simulink model "STM32_IIR_test_script"  (R2018b)
settings: Solver=FixedStepAuto  StartTime=0.0  StopTime=10.0  RelTol=1e-3  EnableMultiTasking=on
libraries: stm32f769ilib x2
settings Model: Creator=hpong  LastModifiedBy=hpong
settings OptimizationCC: EnhancedBackFolding=on  PassReuseOutputArgsAs=Individual arguments  MaxStackSize=64  OptimizeBlockOrder=speed  DifferentSizesBufferReuse=on  OptimizationCustomize=off
settings DebuggingCC: ParameterTunabilityLossMsg=error  LibraryContextMissingDiagnostic=none
settings HardwareCC: ProdBitPerPointer=32  ProdBitPerSizeT=32  ProdBitPerPtrDiffT=32  ProdLargestAtomicInteger=Long  ProdLargestAtomicFloat=Double  ProdWordSize=32  ProdHWDeviceType=ARM Compatible->ARM Cortex
settings SFSimCC: SimUseLocalCustomCode=off  MATLABDynamicMemAlloc=off
settings RTWCC: SystemTargetFile=ert.tlc  HardwareBoard=STM32F769I-Discovery  TemplateMakefile=ert_default_tmf  GenerateReport=on  RTWUseLocalCustomCode=off  Toolchain=GNU Tools for ARM Embedded Processors  IncludeHyperlinkInReport=on  LaunchReport=on  GenerateTraceInfo=on  GenerateTraceReport=on  GenerateTraceReportSl=on  GenerateTraceReportSf=on  GenerateTraceReportEml=on
settings CodeAppCC: ForceParamTrailComments=on  IgnoreCustomStorageClasses=off  OperatorAnnotations=on  SimulinkDataObjDesc=on  SFDataObjDesc=on  InsertBlockDesc=on
settings ERTTargetCC: CodeReplacementLibrary=ARM Cortex-M (CMSIS)

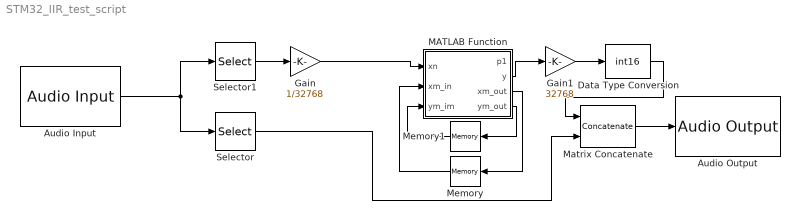
== system STM32_IIR_test_script ==
  Audio Input : stm32f769ilib/Audio Input  InputDevice=LineIn  SamplingFreq=48000  NumCh=2  FrameSize=12
      settings: SourceProductName=Embedded Coder Support Package for STMicroelectronics Discovery Boards  SourceProductBaseCode=STMICRODIS
  Audio Output : stm32f769ilib/Audio Output  OutputDevice=Headphone  SamplingFreq=48000  Volume=65
      settings: SourceProductName=Embedded Coder Support Package for STMicroelectronics Discovery Boards  SourceProductBaseCode=STMICRODIS
  Data Type Conversion : DataTypeConversion  OutDataTypeStr=int16
  Gain : Gain  Gain=1/32768  OutDataTypeStr=double
  Gain1 : Gain  Gain=32768
  MATLAB Function : MATLAB Function  TreatAsAtomicUnit=on
  Matrix Concatenate : Concatenate  Mode=Multidimensional array  ConcatenateDimension=2
  Memory : Memory  InitialCondition="[0  0  0  0  0  0  0  0  0  0  0  0  0  0  0  0  0  0  0  0  0  0  0  0  0  0  ]"  InheritSampleTime=on
  Memory1 : Memory  InitialCondition="[0  0  0  0  0  0  0  0  0  0  0  0  0  0  0  0  0  0  0  0  0  0  0  0  0  0  ]"  InheritSampleTime=on
  Selector : Selector  NumberOfDimensions=2  InputPortWidth=2  IndexOptions=Select all,Index vector (dialog)  Indices=1,2  OutputSizes=1,1
  Selector1 : Selector  NumberOfDimensions=2  InputPortWidth=2  IndexOptions=Select all,Index vector (dialog)  Indices=1,1  OutputSizes=1,1
  wires:
  Matrix Concatenate/1 -> Audio Output/1
  Audio Input/1 -> Selector1/1, Selector/1
  Selector/1 -> Matrix Concatenate/2
  Selector1/1 -> Gain/1
  Gain1/1 -> Data Type Conversion/1
  MATLAB Function/2(y) -> Gain1/1
  MATLAB Function/3(xm_out) -> Memory/1
  MATLAB Function/4(ym_out) -> Memory1/1
  Memory/1 -> MATLAB Function/2(xm_in)
  Memory1/1 -> MATLAB Function/3(ym_im)
  Data Type Conversion/1 -> Matrix Concatenate/1
  Gain/1 -> MATLAB Function/1(xn)

== matlab function STM32_IIR_test_script/MATLAB Function ==
  data: p1 output; xn input; xm_in input; ym_im input; y output; xm_out output; ym_out output
function [p1,y, xm_out, ym_out] = iir_test(xn, xm_in, ym_im)
b = [0.000000000000000990  0.000000000000025742  0.000000000000321780  0.000000000002574243  0.000000000014801897  0.000000000065128345  0.000000000227949209  0.000000000651283454  0.000000001546798204  0.000000003093596408  0.000000005259113893  0.000000007649620208  0.000000009562025260  0.000000010297565665  0.000000009562025260  0.000000007649620208  0.000000005259113893  0.000000003093596408  0.000000001546798204  0.000000000651283454  0.000000000227949209  0.000000000065128345  0.000000000014801897  0.000000000002574243  0.000000000000321780  0.000000000000025742  0.000000000000000990  ];
a = [1.000000000000000000  -15.595213999353305212  118.336259655011303948  -581.126161991364142523  2072.722057324465822603  -5713.051008179993004887  12642.818748640363992308  -23041.152691919291100930  35198.581434592539153527  -45642.355669735632545780  50690.606897819838195574  -48519.739257347500824835  40189.495496968629595358  -28872.161761595212738030  17999.537219242418359499  -9727.415527088094677310  4544.621559022650217230  -1827.116502547159143433  627.852857272126243515  -182.658410835229403801  44.401873881118547160  -8.855309548781658435  1.411663579417976599  -0.173017303518070875  0.015311280179496215  -0.000871047933122563  0.000023926742299957  ];

p1 = 1;
y=ones(12,1,'double');
xm = xm_in; %4*1
ym = ym_im; %4*1
for n=1:12
%     y(n) = b(1)*xn(n) + b(2)*xm(1) + b(3)*xm(2)+ b(4)*xm(3) + b(5)*xm(4) - a(2)*ym(1) - a(3)*ym(2) - a(4)*ym(3) - a(5)*ym(4);
    y(n) = b(1)*xn(n);
    for nn=1:length(b)-1
    y(n) = y(n) +  b(nn+1)*xm(nn) -  a(nn+1)*ym(nn); 
    end
  for i=length(b)-2:-1:1
     xm(i+1) = xm(i); 
     ym(i+1) = ym(i);
  end
  xm(1) = xn(n);
  ym(1) = y(n);
end
xm_out = xm;
ym_out = ym;
end
p1 = 0;
